simulink model "ed3"  (R2023b)
settings: Solver=VariableStepAuto  StartTime=0.0  StopTime=1  RelTol=1e-3
libraries: spsIGBTLib x6, spsAsynchronousMachineSIUnitsLib x1, spsDCVoltageSourceLib x1, spsVoltageMeasurementLib x1, sps_lib x1
settings SolverCC: ZeroCrossAlgorithm=Adaptive
settings DebuggingCC: IgnoredZcDiagnostic=none

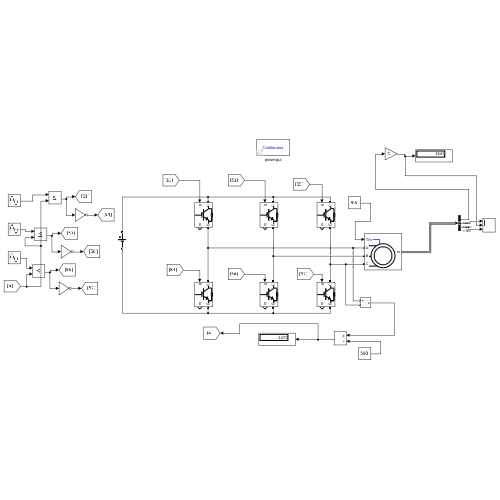
[thumbnail: Simulink's stored preview of the top-level diagram]
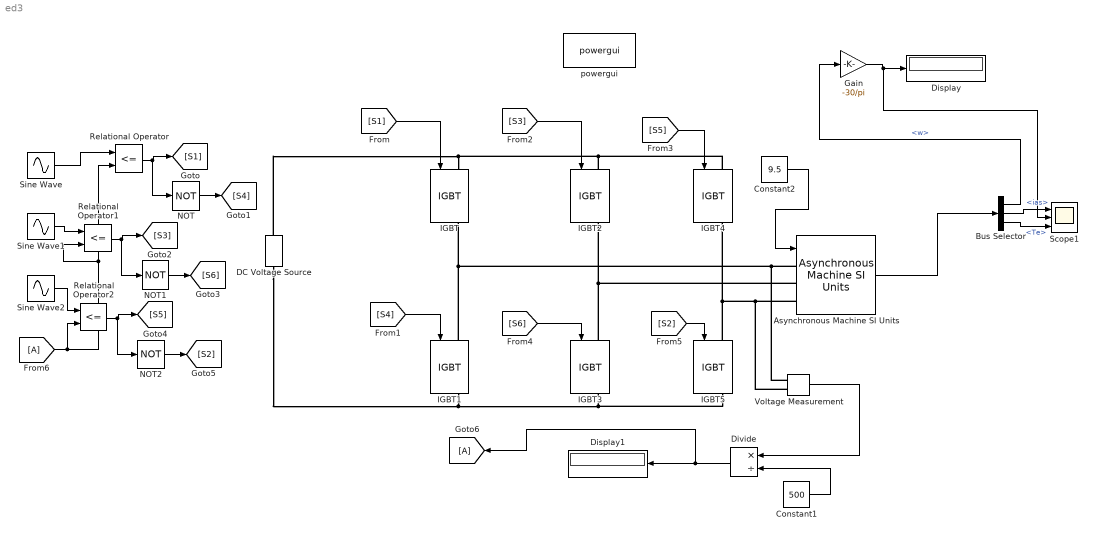
== system ed3 ==
  Asynchronous Machine SI Units : spsAsynchronousMachineSIUnitsLib/Asynchronous Machine SI Units  RotorType=Squirrel-cage  PresetModel="15:  5.4 HP (4KW)   400 V  50Hz 1430 RPM"  MechanicalLoad=Torque Tm  ShowDetailedParameters=on  ReferenceFrame=Synchronous  Units=SI  MeasurementBus=on  NominalParameters=[4000 400 50]  VoltageRatio=0.5  Stator=[1.405 0.005839]  Rotor=[1.395 0.005839]  Cage1=[0.4155 0.002066]  Cage2=[0.4168 0.0003495]  Lm=0.1722  Mechanical=[0.0131 0.002985 2]  PolePairs=2  InitialConditions=[0 0 0 0 0 0 0 0]  SimulateSaturation=off  Saturation=[14.03593122, 27.81365428, 53.79336849, 72.68890987, 97.98006896, 148.6815601, 215.7428561, 302.9841135, 428.7778367 ; 230, 322, 414, 460, 506, 552, 598, 644, 690]  LoadFlowParameters=1492000  TsPowergui=0  TsBlock=-1  IterativeModel=Trapezoidal non iterative  IterativeDiscreteModel=Trapezoidal non iterative  Pmec=1.492e+006
  Bus Selector : BusSelector  OutputSignals=w,ias,Te
  Constant1 : Constant  Value=500
  Constant2 : Constant  Value=9.5
  DC Voltage Source : spsDCVoltageSourceLib/DC Voltage Source  Amplitude=400  Measurements=Voltage
  Display : Display
  Display1 : Display
  Divide : Product  Inputs=*/  RndMeth=Zero  SaturateOnIntegerOverflow=on
  From6 : From
  Gain : Gain  Gain=-30/pi
  Goto6 : Goto
  IGBT{,1..5} (6 alike) : spsIGBTLib/IGBT  Ron=0.001  Lon=0  Vf=1  Tf=1e-6  Tt=2e-6  IC=0  Rs=1e5  Cs=inf  Measurements=on
  NOT : Logic  Operator=NOT  IconShape=distinctive  AllPortsSameDT=off  OutDataTypeStr=boolean
  NOT1 : Logic  Operator=NOT  IconShape=distinctive  AllPortsSameDT=off  OutDataTypeStr=boolean
  NOT2 : Logic  Operator=NOT  IconShape=distinctive  AllPortsSameDT=off  OutDataTypeStr=boolean
  Relational Operator : RelationalOperator  Operator=<=  OutDataTypeStr=boolean  RndMeth=Simplest  InputSameDT=off
  Relational Operator1 : RelationalOperator  Operator=<=  OutDataTypeStr=boolean  RndMeth=Simplest  InputSameDT=off
  Relational Operator2 : RelationalOperator  Operator=<=  OutDataTypeStr=boolean  RndMeth=Simplest  InputSameDT=off
  Scope1 : Scope  NumInputPorts=3
  Sine Wave : Sin  Frequency=50*2*pi  SampleTime=0
  Sine Wave1 : Sin  Frequency=50*2*pi  Phase=120*(pi/180)  SampleTime=0
  Sine Wave2 : Sin  Frequency=50*2*pi  Phase=240*(pi/180)  SampleTime=0
  Voltage Measurement : spsVoltageMeasurementLib/Voltage Measurement  PhasorSimulation=off  OutputType=Complex  PSBequivalent=0
  powergui : sps_lib/powergui  Priority=1  SimulationMode=Continuous  SampleTime=50e-6  frequency=60  Iterations=50  frequencyindice=50  Pbase=100e6  ErrMax=1e-4  UnitsV=kV  UnitsW=MW  buscounter=0  FunctionMessages=off  echomessages=off  EnableUseOfTLC=off  CurrentSourceSwitches=off  DisableSnubberDevices=off  DisableRonSwitches=off  DisableVfSwitches=off  DisplayEquations=off  AutomaticDiscreteSolvers=off  SolverType=Tustin/Backward Euler (TBE)  Interpol=off  ExternalGateDelay=off  methode=off  Ts=100  x0status=blocks  SPID=on  SwTol=0  HookPort=off  NonlinearTolerance=1e-4  nMaxIteration=100  ContinueOnMaxIteration=off  RestoreLinks=warning  ResistiveCurrentMeasurement=off  Frange=[0:2:500]  Ylog=off  Xlog=on  ShowGrid=off  save=off  variable=ZData  structure=0  ZoomFFT=off  StartTime=0.0  cycles=1  DisplayStyle=1  fundamental=60  FreqAxis=off  MaxFrequency=1000  frequencyindicesteady=1  RmsSteady=1  display=off
  wires:
  Asynchronous Machine SI Units/1 -> Bus Selector/1
  Sine Wave/1 -> Relational Operator/1
  From6/1 -> Relational Operator1/2, Relational Operator/2, Relational Operator2/2
  Relational Operator/1 -> NOT/1, [S1]
  NOT/1 -> [S4]
  [S1] -> IGBT/1
  [S4] -> IGBT1/1
  Relational Operator1/1 -> NOT1/1, [S3]
  NOT1/1 -> [S6]
  Sine Wave1/1 -> Relational Operator1/1
  Relational Operator2/1 -> NOT2/1, [S5]
  NOT2/1 -> [S2]
  Sine Wave2/1 -> Relational Operator2/1
  [S6] -> IGBT3/1
  [S3] -> IGBT2/1
  [S5] -> IGBT4/1
  [S2] -> IGBT5/1
  Gain/1 -> Scope1/2, Display/1
  Bus Selector/2 -> Scope1/1  "<ias>"
  Bus Selector/3 -> Scope1/3  "<Te>"
  Bus Selector/1 -> Gain/1  "<w>"
  Voltage Measurement/1 -> Divide/1
  Constant1/1 -> Divide/2
  Divide/1 -> Goto6/1, Display1/1
  Constant2/1 -> Asynchronous Machine SI Units/1
  connections:
  IGBT1/LConn1 -- Voltage Measurement/LConn1 -- Asynchronous Machine SI Units/LConn1 -- IGBT/RConn1
  IGBT3/LConn1 -- Asynchronous Machine SI Units/LConn2 -- IGBT2/RConn1
  IGBT5/LConn1 -- Voltage Measurement/LConn2 -- Asynchronous Machine SI Units/LConn3 -- IGBT4/RConn1
  DC Voltage Source/RConn1 -- IGBT4/LConn1 -- IGBT2/LConn1 -- IGBT/LConn1
  IGBT5/RConn1 -- DC Voltage Source/LConn1 -- IGBT1/RConn1 -- IGBT3/RConn1
